simulink model "mini_project_v2"  (R2024a)
settings: Solver=VariableStepAuto  StartTime=0.0  StopTime=10.0  RelTol=1e-3
libraries: c280xlib x2, simulink x1
settings Model: Creator=surbh  LastModifiedBy=surbh

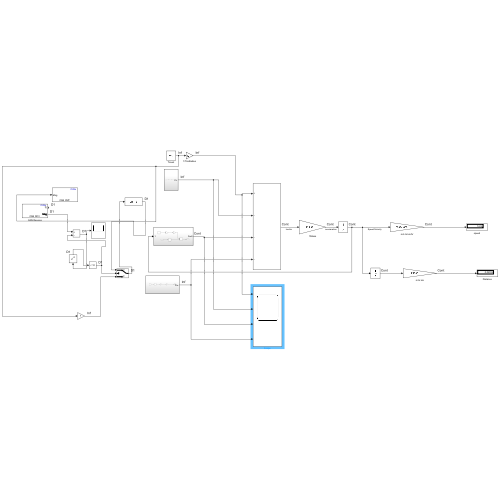
[thumbnail: Simulink's stored preview of the top-level diagram]
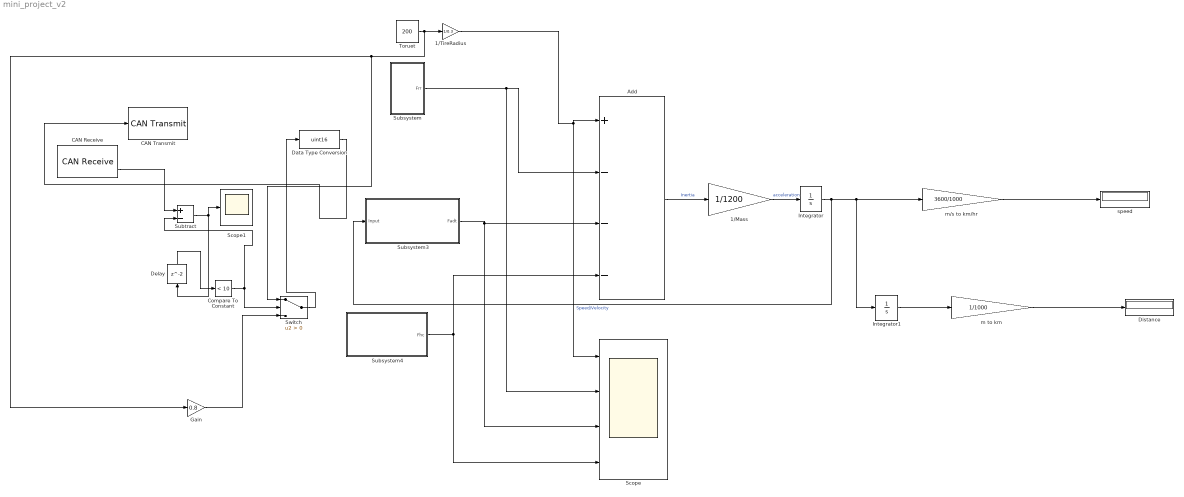
== system mini_project_v2 ==
  1/Mass : Gain  Gain=1/1200
  1/TireRadius : Gain  Gain=1/0.3
  Add : Sum  Inputs=+---
  CAN Receive : c280xlib/CAN Receive  chipFamily=C280x  useModule=CAN_A  mailboxNo=0  messageID=bin2dec('111000111')  messageType=Standard (11-bit identifier)  enableAcceptanceFiltering=off  messageIDMask=0  sampleTime=1  dataType=uint16  outputAction=Output last received values  initValue=0  outputMessageID=off  outputMessageLength=off  outputMessageTimeStamp=off  postInterrupt=off  interruptLine=0
  CAN Transmit : c280xlib/CAN Transmit  chipFamily=C280x  useModule=CAN_A  mailboxNo=1  messageID=bin2dec('111000111')  messageType=Standard (11-bit identifier)  enableBlockingMode=off  postInterrupt=off  interruptLine=0
  Compare To Constant : simulink/Logic and Bit Operations/Compare To Constant  relop=<  const=10  OutDataTypeStr=boolean
  Data Type Conversion : DataTypeConversion  OutMin=0  OutMax=65535  OutDataTypeStr=uint16  SaturateOnIntegerOverflow=off  RndMeth=Floor
  Delay : Delay
  Distance : Display
  Gain : Gain  Gain=0.8
  Integrator : Integrator
  Integrator1 : Integrator
  Scope : Scope  NumInputPorts=4
  Scope1 : Scope
  Subsystem : Subsystem
  Subsystem3 : Subsystem
  Subsystem4 : Subsystem
  Subtract : Sum  Inputs=+-  OutMin=0  OutMax=65535  OutDataTypeStr=uint16  AccumDataTypeStr=uint16
  Switch : Switch  Criteria=u2 > Threshold  SaturateOnIntegerOverflow=off  InputSameDT=off
  Toruet : Constant  Value=200
  m to km : Gain  Gain=1/1000
  m/s to km/hr : Gain  Gain=3600/1000
  speed : Display
  wires:
  Subsystem/1(Frr) -> Scope/2, Add/2
  Integrator/1 -> Integrator1/1, m/s to km/hr/1, Subsystem3/1(Input)  "Speed/Velocity"
  Subsystem3/1(Fadt) -> Add/3, Scope/3
  Subsystem4/1(Fhc) -> Add/4, Scope/4
  Add/1 -> 1/Mass/1  "Inertia"
  1/TireRadius/1 -> Scope/1, Add/1
  1/Mass/1 -> Integrator/1  "acceleration"
  m/s to km/hr/1 -> speed/1
  Integrator1/1 -> m to km/1
  m to km/1 -> Distance/1
  CAN Receive/2 -> Subtract/1
  Compare To Constant/1 -> Subtract/2, Switch/2
  Toruet/1 -> Switch/1, Gain/1, 1/TireRadius/1
  Gain/1 -> Switch/3
  Switch/1 -> Data Type Conversion/1
  Data Type Conversion/1 -> CAN Transmit/1
  Subtract/1 -> Scope1/1, Delay/1
  Delay/1 -> Compare To Constant/1

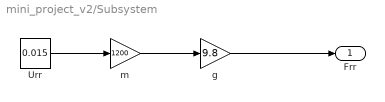
== system mini_project_v2/Subsystem ==
  Urr : Constant  Value=0.015
  g : Gain  Gain=9.8
  m : Gain  Gain=1200
  Frr : Outport
  wires:
  Urr/1 -> m/1
  m/1 -> g/1
  g/1 -> Frr/1

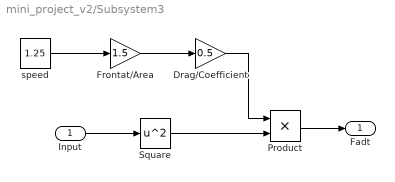
== system mini_project_v2/Subsystem3 ==
  Input : Inport
  Drag/Coefficient : Gain  Gain=0.5
  Frontat/Area : Gain  Gain=1.5
  Product : Product
  Square : Math  Operator=square
  speed : Constant  Value=1.25
  Fadt : Outport
  wires:
  Input/1 -> Square/1
  Drag/Coefficient/1 -> Product/1
  speed/1 -> Frontat/Area/1
  Frontat/Area/1 -> Drag/Coefficient/1
  Product/1 -> Fadt/1
  Square/1 -> Product/2

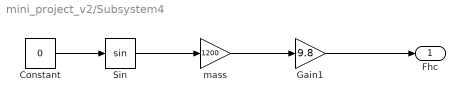
== system mini_project_v2/Subsystem4 ==
  Constant : Constant  Value=0
  Gain1 : Gain  Gain=9.8
  Sin : Trigonometry
  mass : Gain  Gain=1200
  Fhc : Outport
  wires:
  Constant/1 -> Sin/1
  Gain1/1 -> Fhc/1
  Sin/1 -> mass/1
  mass/1 -> Gain1/1
